simulink model "ArduinoMultithreadTest"  (R2014a)
settings: Solver=ode3  SolverMode=SingleTasking  StartTime=0.0  StopTime=10.0  RelTol=1e-3
libraries: arduinolib x2
settings Model: ExtModeTrigDuration=2  Creator=beaverl  LastModifiedBy=beaverl
settings OptimizationCC: OptimizeModelRefInitCode=on  LifeSpan=1
settings DebuggingCC: UnderspecifiedInitializationDetection=Classic  SolverPrmCheckMsg=none
settings HardwareCC: ProdBitPerInt=16  ProdBitPerPointer=8  ProdIntDivRoundTo=Zero  ProdEndianess=LittleEndian  ProdWordSize=8  ProdHWDeviceType=Atmel->AVR
settings RTWCC: SystemTargetFile=realtime.tlc  GenerateMakefile=off  TemplateMakefile=realtime.tmf  Description=Run on Target Hardware  RTWVerbose=off  ProcessScript=realtime_make_rtw_hook
settings STFCustomTargetCC: TargetLibSuffix=.a  GenerateSampleERTMain=on  ConcurrentExecutionCompliant=off  GeneratePreprocessorConditionals=Use local settings  ERTCustomFileBanners=on  SupportNonInlinedSFcns=off  SupportVariableSizeSignals=on  MATLABClassNameForMDSCustomization=Simulink.SoftwareTarget.ERTCustomization  GRTInterface=off  SystemTargetFile=realtime.tlc
settings ERTTargetCC: CombineOutputUpdateFcns=off  SupportContinuousTime=on  SupportVariableSizeSignals=on  ExtModeTransport=3  ExtModeMexFile=ext_serial_win32_comm  ExtModeMexArgs=0 1 9600  ERTSrcFileBannerTemplate=realtime_code_template.cgt  ERTHdrFileBannerTemplate=realtime_code_template.cgt  ERTDataSrcFileTemplate=realtime_code_template.cgt  ERTDataHdrFileTemplate=realtime_code_template.cgt  ERTCustomFileTemplate=realtime_file_process.tlc

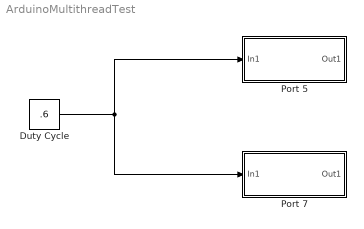
== system ArduinoMultithreadTest ==
  Duty Cycle : Constant  Value=.6
  Port 5 : Subsystem
  Port 7 : Subsystem
  wires:
  Duty Cycle/1 -> Port 7/1(In1), Port 5/1(In1)

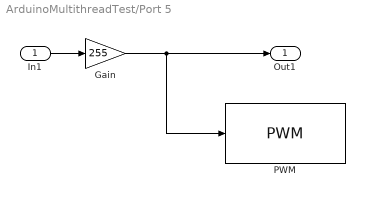
== system ArduinoMultithreadTest/Port 5 ==
  In1 : Inport
  Gain : Gain  Gain=255
  PWM : arduinolib/PWM  pinNumber=5
  Out1 : Outport
  wires:
  In1/1 -> Gain/1
  Gain/1 -> PWM/1, Out1/1

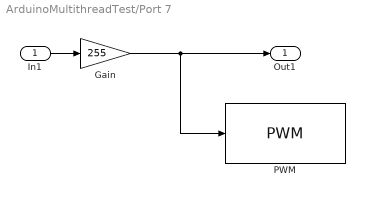
== system ArduinoMultithreadTest/Port 7 ==
  In1 : Inport
  Gain : Gain  Gain=255
  PWM : arduinolib/PWM  pinNumber=7
  Out1 : Outport
  wires:
  In1/1 -> Gain/1
  Gain/1 -> PWM/1, Out1/1
